simulink model "dspautoscale"  (Simulink 8.3)
settings: Solver=FixedStepDiscrete  SolverMode=SingleTasking  StartTime=0.0  StopTime=inf  RelTol=1e-3
model workspace (MATLAB code in the model file):
  | FracPeriod=0.5; % fraction of period of sinusoid that we will match
  | N=25; %Total number points for estimate
  | Npoly=2; % Order of polynomial to use in fitting
  | Duration = 2; % Total length of observation window
  | Ts = Duration / N; % Sample interval
undefined symbols (not defined in the file or in its folder): NN
libraries: dspsrcs4 x2, dspmtrx3 x2, dspsolvers x1, dspmisc x1, dspfactors x1, dsppolyfun x1
CloseFcn:
  | clear FixPtSimRanges;
settings Model: DataTypeOverride=Double  MinMaxOverflowLogging=MinMaxAndOverflow  Creator=The MathWorks Inc.  ExtModeAutoUpdateStatusClock=off
settings DataIOCC: SaveOutput=off  SignalLogging=off  SaveTime=off
settings OptimizationCC: InlineParams=on  ExpressionDepthLimit=2147483647  InitFltsAndDblsToZero=on  EfficientMapNaN2IntZero=off
settings DebuggingCC: SignalResolutionControl=TryResolveAllWithWarning  SolverPrmCheckMsg=none  FcnCallInpInsideContextMsg=UseLocalSettings  StrictBusMsg=Warning
settings HardwareCC: ProdHWDeviceType=ASIC/FPGA  TargetBitPerLong=64  TargetBitPerPointer=64  TargetLongLongMode=on  TargetEndianess=LittleEndian  TargetWordSize=64  TargetHWDeviceType=MATLAB Host  ProdEqTarget=off
settings SFSimCC: SimParseCustomCode=off
settings RTWCC: GenerateReport=on  LaunchReport=on
settings GRTTargetCC: TargetFcnLib=ansi_tfl_tmw_new.mat

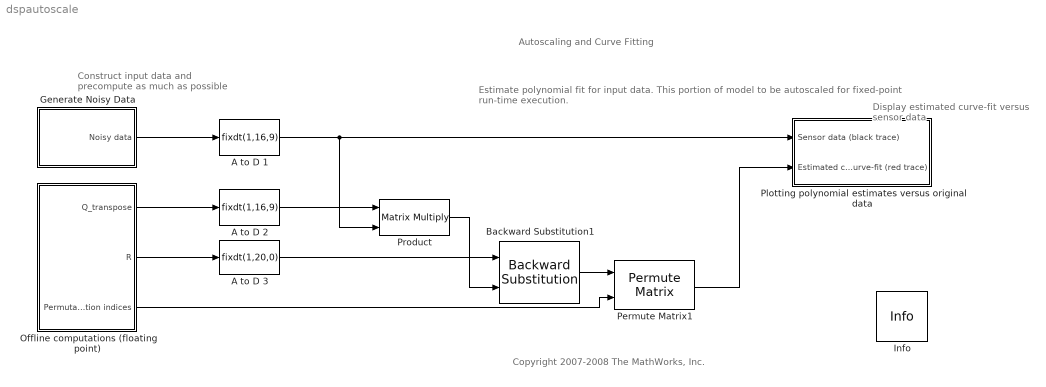
== system dspautoscale ==
  note: Autoscaling and Curve Fitting
  note: Construct input data
      | and precompute as much
      | as possible
  note: Estimate polynomial fit for input data.
      | This portion of model to be autoscaled for fixed-point run-time execution.
  note: Display estimated curve-fit
      | versus sensor data
  note: Copyright 2007-2008 The MathWorks, Inc.
  A to D 1 : DataTypeConversion  OutDataTypeStr=fixdt(1,16,9)  RndMeth=Nearest
  A to D 2 : DataTypeConversion  OutDataTypeStr=fixdt(1,16,9)  RndMeth=Nearest
  A to D 3 : DataTypeConversion  OutDataTypeStr=fixdt(1,20,0)  RndMeth=Nearest
  Backward Substitution1 : dspsolvers/Backward Substitution  Unit=off  RealDiag=on  outputMode=Binary point scaling  outputWordLength=16  outputFracLength=15  outputDataTypeStr=fixdt(1,16,15)  outputLastDataTypeStr=fixdt(1,16,15)  outputMin=[]  outputMax=[]  accumMode=Binary point scaling  accumWordLength=32  accumFracLength=30  accumDataTypeStr=fixdt(1,32,30)  accumLastDataTypeStr=fixdt(1,32,30)  prodOutputMode=Binary point scaling  prodOutputWordLength=32  prodOutputFracLength=30  prodOutputDataTypeStr=fixdt(1,32,30)  prodOutputLastDataTypeStr=fixdt(1,32,30)  roundingMode=Floor  overflowMode=off
  Generate Noisy Data : Subsystem
  Info : dspmisc/Info  SystemSampleTime=-1
  Offline computations (floating point) : Subsystem
  Permute Matrix1 : dspmtrx3/Permute Matrix  mode=Rows  ZeroOneIdxMode=One-based  errmode=Clip index  checkDims=off
  Plotting polynomial estimates versus original data : Subsystem
  Product : Product  Multiplication=Matrix(*)  OutDataTypeStr=fixdt(1,32,31)  RndMeth=Zero
  wires:
  Generate Noisy Data/1(Noisy data) -> A to D 1/1
  A to D 1/1 -> Plotting polynomial estimates versus original data/1(Sensor data (black trace)), Product/2
  A to D 3/1 -> Backward Substitution1/1
  Offline computations (floating point)/2(R) -> A to D 3/1
  Offline computations (floating point)/1(Q_transpose) -> A to D 2/1
  Product/1 -> Backward Substitution1/2
  Backward Substitution1/1 -> Permute Matrix1/1
  A to D 2/1 -> Product/1
  Permute Matrix1/1 -> Plotting polynomial estimates versus original data/2(Estimated curve-fit (red trace))
  Offline computations (floating point)/3(Permutation indices) -> Permute Matrix1/2

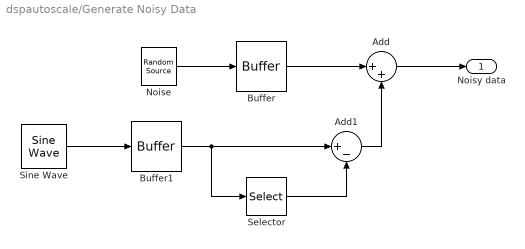
== system dspautoscale/Generate Noisy Data ==
  Add : Sum  Inputs=|++
  Add1 : Sum  Inputs=|+-
  Buffer : Buffer  N=N  V=N-1  TreatMby1Signals=One channel
  Buffer1 : Buffer  N=N  V=N-1  TreatMby1Signals=One channel
  Noise : dspsrcs4/Random Source  SrcType=Gaussian  NormMethod=Ziggurat  CltLength=12  MinVal=0  MaxVal=1  MeanVal=0  VarVal=0.1  RepMode=Repeatable  rawSeed=1  IsInherit=off  SampMode=Discrete  SampTime=Ts  SampFrame=1  DataType=Double  OutComplex=Real
  Selector : Selector  NumberOfDimensions=2  InputPortWidth=3  IndexOptions=Index vector (dialog),Select all  Indices=1,[N+2-NN]  OutputSizes=1,NN
  Sine Wave : dspsrcs4/Sine Wave  Amplitude=1  Frequency=FracPeriod/(N*Ts)  Phase=0  SampleMode=Discrete  OutComplex=Real  CompMethod=Trigonometric fcn  TableSize=Speed  SampleTime=Ts  SamplesPerFrame=1  ResetState=Restart at time zero  dataType=double  wordLen=16  udDataType=sfix(16)  fracBitsMode=Best precision  numFracBits=15  OutDataTypeStr=double  LastOutDataTypeStr=double
  Noisy data : Outport
  wires:
  Noise/1 -> Buffer/1
  Add/1 -> Noisy data/1
  Buffer1/1 -> Selector/1, Add1/1
  Buffer/1 -> Add/1
  Selector/1 -> Add1/2
  Add1/1 -> Add/2
  Sine Wave/1 -> Buffer1/1

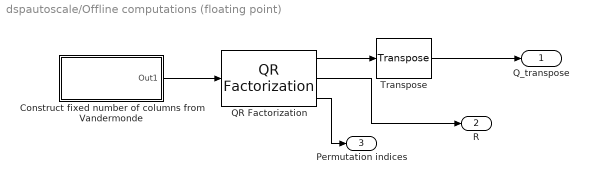
== system dspautoscale/Offline computations (floating point) ==
  Construct fixed number of columns from Vandermonde : Subsystem  mask{nsamps=N, tsamp=Ts, npoly=Npoly}
      mask prompts: nsamps "Number of samples:"; tsamp "Sample time:"; npoly "Polynomial order:"
      mask init:
      | v=[0:tsamp:((nsamps-1)*tsamp)]';
      | polymatrix = v;
      | for i=2:npoly
      |     polymatrix = [v.^i polymatrix];
      | end
  QR Factorization : dspfactors/QR Factorization  outputSize=Economy
  Transpose : dspmtrx3/Transpose  Hermitian=off  overflowFlag=off
  Q_transpose : Outport
  R : Outport  Port=2
  Permutation indices : Outport  Port=3
  wires:
  QR Factorization/1 -> Transpose/1
  Construct fixed number of columns from Vandermonde/1(Out1) -> QR Factorization/1
  Transpose/1 -> Q_transpose/1
  QR Factorization/3 -> Permutation indices/1
  QR Factorization/2 -> R/1

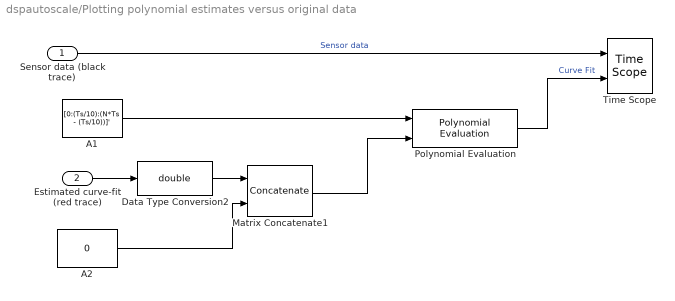
== system dspautoscale/Plotting polynomial estimates versus original data ==
  Sensor data (black trace) : Inport
  Estimated curve-fit (red trace) : Inport  Port=2
  A1 : Constant  Value=[0:(Ts/10):(N*Ts - (Ts/10))]'  VectorParams1D=off  OutDataTypeStr=double
  A2 : Constant  Value=0  VectorParams1D=off  OutDataTypeStr=double
  Data Type Conversion2 : DataTypeConversion  OutDataTypeStr=double  RndMeth=Nearest
  Matrix Concatenate1 : Concatenate  ConcatenateDimension=2
  Polynomial Evaluation : dsppolyfun/Polynomial Evaluation  useConstCoeffs=off  constCoeffs=[5 4 3 2 1]
  Time Scope : TimeScope  NumInputPorts=2  DefaultConfigurationName=spbscopes.TimeScopeBlockCfg  ScopeSpecification=DataTag1
  wires:
  Sensor data (black trace)/1 -> Time Scope/1  "Sensor data"
  A1/1 -> Polynomial Evaluation/1
  Matrix Concatenate1/1 -> Polynomial Evaluation/2
  A2/1 -> Matrix Concatenate1/2
  Estimated curve-fit (red trace)/1 -> Data Type Conversion2/1
  Data Type Conversion2/1 -> Matrix Concatenate1/1
  Polynomial Evaluation/1 -> Time Scope/2  "Curve Fit"

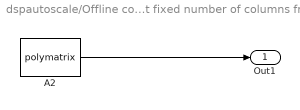
== system dspautoscale/Offline computations (floating point)/Construct fixed number of columns from Vandermonde ==
  A2 : Constant  Value=polymatrix  VectorParams1D=off  OutDataTypeStr=double
  Out1 : Outport
  wires:
  A2/1 -> Out1/1
